simulink model "simplified_inverter"  (R2021b)
settings: Solver=ode23tb  StartTime=0.0  StopTime=0.1  MaxStep=10e-6  RelTol=1e-3  EnableMultiTasking=on
libraries: spsVoltageMeasurementLib x9, spsSeriesRLCBranchLib x6, spsControlledVoltageSourceLib x3, spsCurrentMeasurementLib x3, spsThreePhaseSourceLib x1, spspowerguiLib x1
settings Model: Creator=Алексей  LastModifiedBy=alexey
settings SolverCC: ZeroCrossControl=DisableAll  ZeroCrossAlgorithm=Adaptive  AlgebraicLoopSolver=TrustRegion
settings DataIOCC: SaveFormat=Array  SaveOutput=off  SignalLogging=off  DSMLogging=off  SaveTime=off  ReturnWorkspaceOutputs=off
settings OptimizationCC: LifeSpan=inf
settings DebuggingCC: UnderspecifiedInitializationDetection=Classic  MergeDetectMultiDrivingBlocksExec=none  SolverPrmCheckMsg=warning  AllowSymbolicDim=off  SFUnexpectedBacktrackingDiag=warning  SFNoUnconditionalDefaultTransitionDiag=warning  SFExecutionAtInitializationDiag=none  SFMachineParentedDataDiag=warning  ArithmeticOperatorsInVariantConditions=warning
settings HardwareCC: ProdBitPerPointer=32  ProdBitPerSizeT=32  ProdBitPerPtrDiffT=32  ProdLargestAtomicFloat=None  ProdIntDivRoundTo=Undefined  ProdEndianess=Unspecified  ProdWordSize=32  ProdHWDeviceType=32-bit Generic
settings ModelReferenceCC: PropagateSignalLabelsOutOfModel=off
settings SFSimCC: SimUseLocalCustomCode=off  CustomCodeUndefinedFunction=UseInterfaceOnly
settings RTWCC: RTWUseLocalCustomCode=off
settings CodeAppCC: StateflowObjectComments=on
settings GRTTargetCC: TargetLangStandard=C89/C90 (ANSI)  RTWCAPISignals=on  RTWCAPIParams=on
settings ConfigComp: CovMetricSettings=dw  CovSaveCumulativeToWorkspaceVar=on  CovSaveSingleToWorkspaceVar=on  CovExternalEMLEnable=off  CovSFcnEnable=off
settings SimscapeCC: SimscapeNormalizeSystem=off

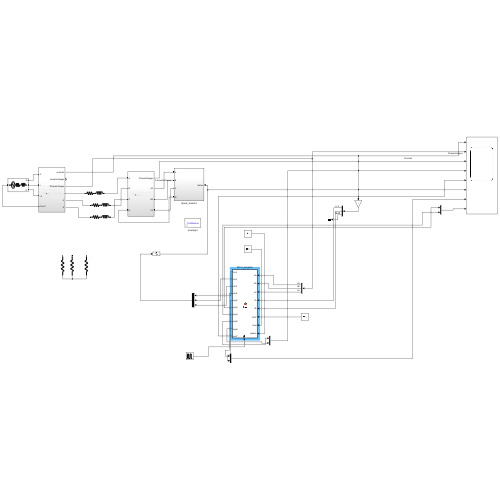
[thumbnail: Simulink's stored preview of the top-level diagram]
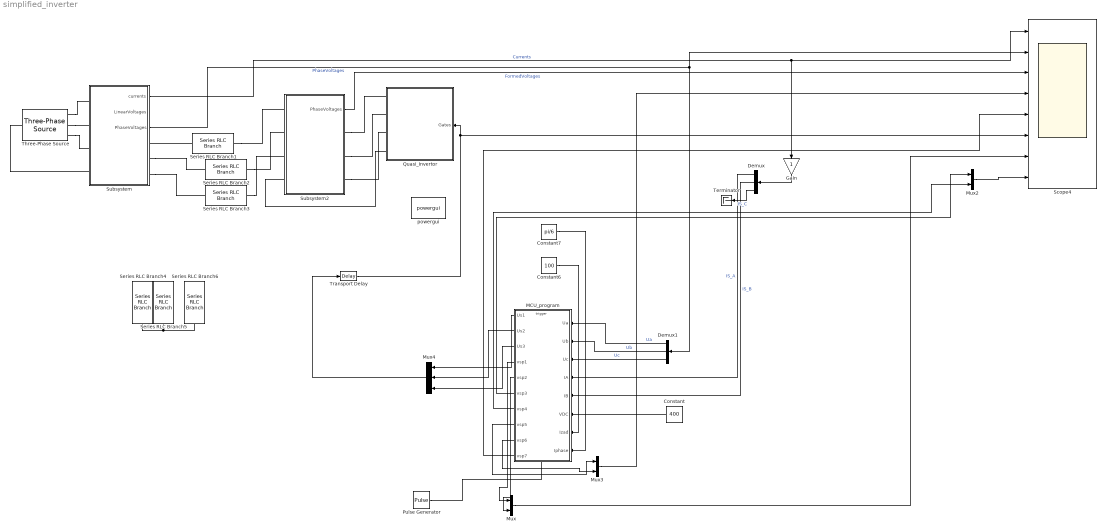
== system simplified_inverter ==
  Constant : Constant  Value=400
  Constant6 : Constant  Value=100
  Constant7 : Constant  Value=pi/6
  Demux : Demux  Outputs=3
  Demux1 : Demux  Outputs=3
  Gain : Gain
  MCU_program : MATLAB Function  TreatAsAtomicUnit=on
  Mux : Mux  Inputs=2
  Mux2 : Mux  Inputs=2
  Mux3 : Mux  Inputs=2
  Mux4 : Mux  Inputs=3
  Pulse Generator : DiscretePulseGenerator  PulseType=Time based  Period=10e-6  PulseWidth=10
  Quasi_Invertor : Subsystem
  Scope4 : Scope  NumInputPorts=8
  Series RLC Branch1 : spsSeriesRLCBranchLib/Series RLC Branch  LConnTagsString=__new0  RConnTagsString=__new0  BranchType=RL  Resistance=0.01  Inductance=50e-6  SetiL0=off  InitialCurrent=0  Capacitance=1e-6  Setx0=off  InitialVoltage=0  Measurements=None
  Series RLC Branch2 : spsSeriesRLCBranchLib/Series RLC Branch  LConnTagsString=__new0  RConnTagsString=__new0  BranchType=RL  Resistance=0.01  Inductance=50e-6  SetiL0=off  InitialCurrent=0  Capacitance=1e-6  Setx0=off  InitialVoltage=0  Measurements=None
  Series RLC Branch3 : spsSeriesRLCBranchLib/Series RLC Branch  LConnTagsString=__new0  RConnTagsString=__new0  BranchType=RL  Resistance=0.01  Inductance=50e-6  SetiL0=off  InitialCurrent=0  Capacitance=1e-6  Setx0=off  InitialVoltage=0  Measurements=None
  Series RLC Branch4 : spsSeriesRLCBranchLib/Series RLC Branch  LConnTagsString=__new0  RConnTagsString=__new0  BranchType=R  Resistance=10  Inductance=500e-6  SetiL0=off  InitialCurrent=0  Capacitance=1e-6  Setx0=off  InitialVoltage=0  Measurements=None
  Series RLC Branch5 : spsSeriesRLCBranchLib/Series RLC Branch  LConnTagsString=__new0  RConnTagsString=__new0  BranchType=R  Resistance=10  Inductance=500e-6  SetiL0=off  InitialCurrent=0  Capacitance=1e-6  Setx0=off  InitialVoltage=0  Measurements=None
  Series RLC Branch6 : spsSeriesRLCBranchLib/Series RLC Branch  LConnTagsString=__new0  RConnTagsString=__new0  BranchType=R  Resistance=10  Inductance=500e-6  SetiL0=off  InitialCurrent=0  Capacitance=1e-6  Setx0=off  InitialVoltage=0  Measurements=None
  Subsystem : Subsystem
  Subsystem2 : Subsystem
  Terminator : Terminator
  Three-Phase Source : spsThreePhaseSourceLib/Three-Phase Source  InternalConnection=Yn  VoltagePhases=on  Voltage=200  PhaseAngle=0  Voltage_phases=[200 200 200]/sqrt(2)  PhaseAngles_phases=[0 -120 +120]  Frequency=500  NonIdealSource=on  SpecifyImpedance=off  Resistance=1e-6  Inductance=30e-9  ShortCircuitLevel=100e6  BaseVoltage=200  XRratio=7  BusType=swing  Pref=10e3  Qref=0  Prefabc=[10e3, 10e3, 10e3]  Qrefabc=[0, 0, 0]  Qmin=-inf  Qmax=inf
  Transport Delay : TransportDelay  DelayTime=1e-6
  powergui : spspowerguiLib/powergui  Priority=1  SimulationMode=Continuous  SampleTime=50e-6  frequency=60  Iterations=50  frequencyindice=500  Pbase=100e6  ErrMax=1e-4  UnitsV=kV  UnitsW=MW  buscounter=0  FunctionMessages=off  echomessages=off  EnableUseOfTLC=off  CurrentSourceSwitches=on  DisableSnubberDevices=off  DisableRonSwitches=off  DisableVfSwitches=off  DisplayEquations=off  AutomaticDiscreteSolvers=off  SolverType=Tustin  Interpol=off  ExternalGateDelay=off  methode=off  Ts=0  x0status=zero  SPID=off  SwTol=0  HookPort=off  NonlinearTolerance=1e-4  nMaxIteration=100  ContinueOnMaxIteration=off  RestoreLinks=warning  ResistiveCurrentMeasurement=off  Frange=[0:2:500]  Ylog=off  Xlog=on  ShowGrid=off  save=off  variable=ZData  structure=SD2  ZoomFFT=on  StartTime=0.7  cycles=10  DisplayStyle=4  fundamental=382  FreqAxis=off  MaxFrequency=50000  frequencyindicesteady=1  RmsSteady=1  display=off
  wires:
  Demux/1 -> MCU_program/4(IA)  "IS_A"
  Demux/2 -> MCU_program/5(IB)  "IS_B"
  MCU_program/5(vsp2) -> Mux/2
  MCU_program/4(vsp1) -> Mux/1
  MCU_program/3(Us3) -> Mux4/3
  Mux4/1 -> Transport Delay/1
  MCU_program/1(Us1) -> Mux4/1
  Pulse Generator/1 -> MCU_program/Trigger
  MCU_program/2(Us2) -> Mux4/2
  Demux/3 -> Terminator/1  "IS_C"
  Demux1/1 -> MCU_program/1(Ua)  "Ua"
  Demux1/2 -> MCU_program/2(Ub)  "Ub"
  Demux1/3 -> MCU_program/3(Uc)  "Uc"
  Subsystem/1(currents) -> Gain/1, Scope4/1  "Currents"
  Mux/1 -> Scope4/7
  Subsystem/3(PhaseVoltages) -> Scope4/2, Demux1/1  "PhaseVoltages"
  MCU_program/7(vsp4) -> Mux2/2
  Constant6/1 -> MCU_program/7(Izad)
  Constant7/1 -> MCU_program/8(Iphase)
  Mux2/1 -> Scope4/8
  MCU_program/6(vsp3) -> Mux2/1
  MCU_program/8(vsp5) -> Mux3/1
  MCU_program/9(vsp6) -> Mux3/2
  Mux3/1 -> Scope4/4
  MCU_program/10(vsp7) -> Scope4/5
  Gain/1 -> Demux/1
  Transport Delay/1 -> Scope4/6, Quasi_Invertor/1(Gates)
  Subsystem2/1(PhaseVoltages) -> Scope4/3  "FormedVoltages"
  Constant/1 -> MCU_program/6(VDC)
  connections:
  Three-Phase Source/RConn1 -- Subsystem/LConn1
  Three-Phase Source/RConn2 -- Subsystem/LConn2
  Three-Phase Source/RConn3 -- Subsystem/LConn3
  Series RLC Branch1/RConn1 -- Subsystem2/LConn1
  Three-Phase Source/LConn1 -- Subsystem/LConn4
  Subsystem2/RConn1 -- Quasi_Invertor/RConn1
  Subsystem2/RConn2 -- Quasi_Invertor/RConn2
  Subsystem2/RConn3 -- Quasi_Invertor/RConn3
  Series RLC Branch2/RConn1 -- Subsystem2/LConn2
  Series RLC Branch3/RConn1 -- Subsystem2/LConn3
  Subsystem2/LConn4 -- Quasi_Invertor/RConn4
  Series RLC Branch4/RConn1 -- Series RLC Branch6/RConn1 -- Series RLC Branch5/RConn1
  Series RLC Branch1/LConn1 -- Subsystem/RConn1
  Subsystem/RConn2 -- Series RLC Branch2/LConn1
  Subsystem/RConn3 -- Series RLC Branch3/LConn1

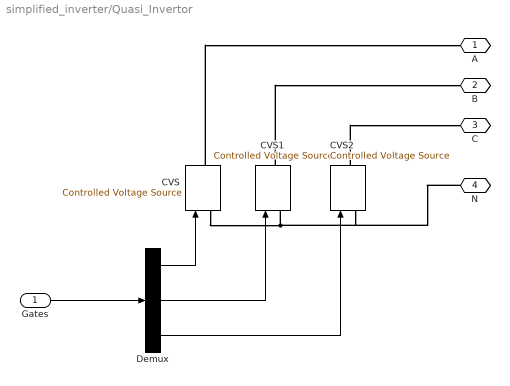
== system simplified_inverter/Quasi_Invertor ==
  Gates : Inport
  CVS : spsControlledVoltageSourceLib/Controlled Voltage Source  Initialize=on  Source_Type=AC  Amplitude=0  Phase=0  Frequency=0  Measurements=None
  CVS1 : spsControlledVoltageSourceLib/Controlled Voltage Source  Initialize=on  Source_Type=AC  Amplitude=0  Phase=0  Frequency=0  Measurements=None
  CVS2 : spsControlledVoltageSourceLib/Controlled Voltage Source  Initialize=on  Source_Type=AC  Amplitude=0  Phase=0  Frequency=0  Measurements=None
  Demux : Demux  Outputs=3
  A : PMIOPort  Side=Right
  B : PMIOPort  Port=2  Side=Right
  C : PMIOPort  Port=3  Side=Right
  N : PMIOPort  Port=4  Side=Right
  wires:
  Demux/1 -> CVS/1
  Demux/2 -> CVS1/1
  Demux/3 -> CVS2/1
  Gates/1 -> Demux/1
  connections:
  CVS1/RConn1 -- B/RConn1
  CVS2/RConn1 -- C/RConn1
  CVS/RConn1 -- A/RConn1
  CVS/LConn1 -- N/RConn1 -- CVS2/LConn1 -- CVS1/LConn1

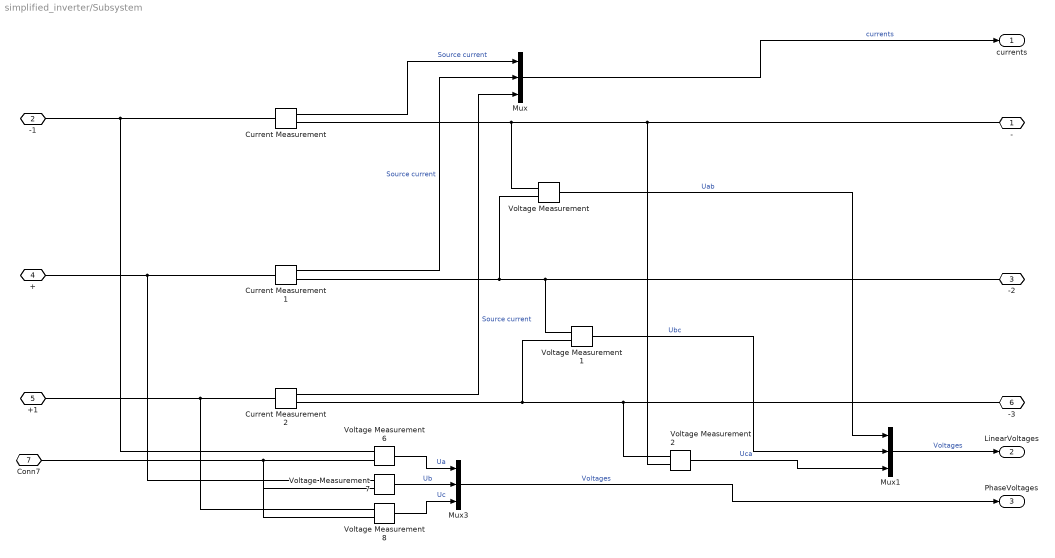
== system simplified_inverter/Subsystem ==
  Current Measurement : spsCurrentMeasurementLib/Current Measurement  PhasorSimulation=off  OutputType=Complex  PSBequivalent=0
  Current Measurement1 : spsCurrentMeasurementLib/Current Measurement  PhasorSimulation=off  OutputType=Complex  PSBequivalent=0
  Current Measurement2 : spsCurrentMeasurementLib/Current Measurement  PhasorSimulation=off  OutputType=Complex  PSBequivalent=0
  Mux : Mux  Inputs=3
  Mux1 : Mux  Inputs=3
  Mux3 : Mux  Inputs=3
  Voltage Measurement{,1..2,6..8} (6 alike) : spsVoltageMeasurementLib/Voltage Measurement  PhasorSimulation=off  OutputType=Complex  PSBequivalent=0
  - : PMIOPort  Side=Right
  -1 : PMIOPort  Port=2  Side=Left
  -2 : PMIOPort  Port=3  Side=Right
  + : PMIOPort  Port=4  Side=Left
  +1 : PMIOPort  Port=5  Side=Left
  -3 : PMIOPort  Port=6  Side=Right
  Conn7 : PMIOPort  Port=7  Side=Left
  currents : Outport
  LinearVoltages : Outport  Port=2
  PhaseVoltages : Outport  Port=3
  wires:
  Current Measurement2/1 -> Mux/3  "Source current"
  Current Measurement1/1 -> Mux/2  "Source current"
  Voltage Measurement1/1 -> Mux1/2  "Ubc"
  Voltage Measurement2/1 -> Mux1/3  "Uca"
  Mux/1 -> currents/1  "currents"
  Voltage Measurement/1 -> Mux1/1  "Uab"
  Current Measurement/1 -> Mux/1  "Source current"
  Mux1/1 -> LinearVoltages/1  "Voltages"
  Mux3/1 -> PhaseVoltages/1  "Voltages"
  Voltage Measurement8/1 -> Mux3/3  "Uc"
  Voltage Measurement6/1 -> Mux3/1  "Ua"
  Voltage Measurement7/1 -> Mux3/2  "Ub"
  connections:
  -1/RConn1 -- Voltage Measurement6/LConn1 -- Current Measurement/LConn1
  Current Measurement1/RConn1 -- Voltage Measurement/LConn2 -- -2/RConn1 -- Voltage Measurement1/LConn1
  Current Measurement/RConn1 -- Voltage Measurement/LConn1 -- Voltage Measurement2/LConn2 -- -/RConn1
  Current Measurement2/RConn1 -- Voltage Measurement2/LConn1 -- -3/RConn1 -- Voltage Measurement1/LConn2
  Voltage Measurement6/LConn2 -- Voltage Measurement8/LConn2 -- Voltage Measurement7/LConn2 -- Conn7/RConn1
  +1/RConn1 -- Voltage Measurement8/LConn1 -- Current Measurement2/LConn1
  +/RConn1 -- Voltage Measurement7/LConn1 -- Current Measurement1/LConn1

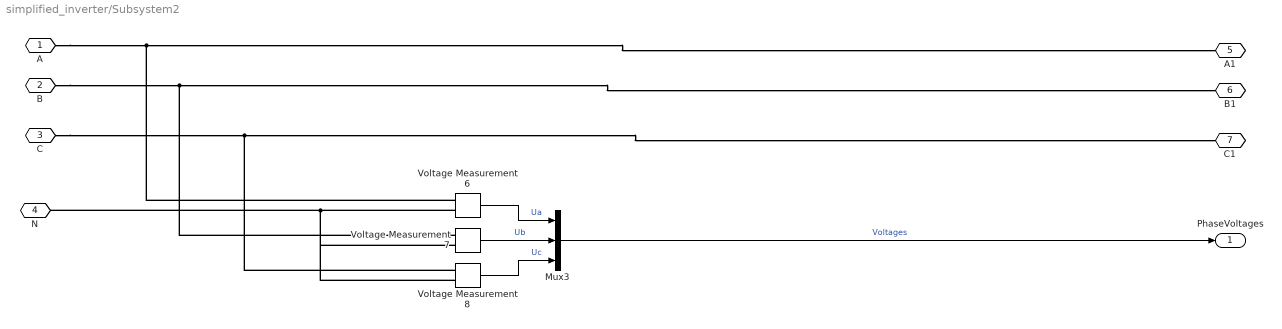
== system simplified_inverter/Subsystem2 ==
  Mux3 : Mux  Inputs=3
  Voltage Measurement6 : spsVoltageMeasurementLib/Voltage Measurement  PhasorSimulation=off  OutputType=Complex  PSBequivalent=0
  Voltage Measurement7 : spsVoltageMeasurementLib/Voltage Measurement  PhasorSimulation=off  OutputType=Complex  PSBequivalent=0
  Voltage Measurement8 : spsVoltageMeasurementLib/Voltage Measurement  PhasorSimulation=off  OutputType=Complex  PSBequivalent=0
  A : PMIOPort  Side=Left
  B : PMIOPort  Port=2  Side=Left
  C : PMIOPort  Port=3  Side=Left
  N : PMIOPort  Port=4  Side=Left
  A1 : PMIOPort  Port=5  Side=Right
  B1 : PMIOPort  Port=6  Side=Right
  C1 : PMIOPort  Port=7  Side=Right
  PhaseVoltages : Outport
  wires:
  Voltage Measurement7/1 -> Mux3/2  "Ub"
  Voltage Measurement6/1 -> Mux3/1  "Ua"
  Voltage Measurement8/1 -> Mux3/3  "Uc"
  Mux3/1 -> PhaseVoltages/1  "Voltages"
  connections:
  Voltage Measurement7/LConn2 -- Voltage Measurement8/LConn2 -- Voltage Measurement6/LConn2 -- N/RConn1
  Voltage Measurement8/LConn1 -- C1/RConn1 -- C/RConn1
  Voltage Measurement6/LConn1 -- A1/RConn1 -- A/RConn1
  Voltage Measurement7/LConn1 -- B1/RConn1 -- B/RConn1

== matlab function simplified_inverter/MCU_program ==
  data: Ua input; Ub input; Uc input; IA input; IB input; Us1 output; Us2 output; Us3 output; vsp1 output; vsp2 output; vsp3 output; vsp4 output; VDC input; Izad input; Iphase input; vsp5 output; vsp6 output; vsp7 output
  events: trigger input RISING_EDGE_EVENT
function [Us1,Us2,Us3,vsp1,vsp2,vsp3,vsp4,vsp5,vsp6,vsp7] = fcn(Ua,Ub,Uc,IA,IB,VDC, Izad, Iphase)
%время 1/2 ШИМ периода
dt = 10e-6;

kuqp = 10;
kuqi = 1000;

kudp = 10;
kudi = 1000;






persistent Uqint;
if isempty(Uqint)
    Uqint=0;
end 
persistent Udint;
if isempty(Udint)
    Udint=0;
end 


Ialfa = -IA;
Ibeta = -(2*IB+IA)/sqrt(3);
I_ampl = sqrt(Ialfa^2+Ibeta^2);

Ualfa = Ua;
Ubeta = (2*Ub+Ua)/sqrt(3);

U_ampl = sqrt(Ualfa^2+Ubeta^2);
teta=acos(Ualfa/U_ampl)*sign(Ubeta)+(sign(Ubeta)-1)*(-pi);



%реальные значения токов Id и Iq, полученные через  угол и оси альфа,бета 
Iact = Ialfa*cos(teta)+Ibeta*sin(teta);
Iact = -Iact; %Перевод в систему координат инвертора - для него поглощается активный ток сети
Ireact = Ibeta*cos(teta)-Ialfa*sin(teta); 

Ireact_zad = -Izad * sin(Iphase);
%ПИ-регулятор для напряжения по оси Ку
direact = Ireact_zad-Ireact;
Uqpr = direact*kuqp;
Uqint=Uqint+direact*kuqi*dt;


Iact_zad = Izad * cos(Iphase);
%ПИ-регулятор для напряжения по оси Дэ
diact = Iact_zad-Iact;
Udpr = diact*kudp;
Udint=Udint+diact*kudi*dt;

Um = (2/3)*VDC/sqrt(Uqpr^2+Udpr^2)*0.85;

if(Um<1)
  Uqpr = Uqpr*Um;
  Udpr = Udpr*Um;
end

  
U_q=Uqpr+Uqint;                    
U_d=Udpr+Udint;


%U_q = 0;
U_d = -U_d;



Ua0=U_d*cos(teta)-U_q*sin(teta);
Ub0=U_d*sin(teta)+U_q*cos(teta);
vrefa=sqrt(Ua0^2+Ub0^2);
tetaV = acos(Ua0/vrefa)*sign(Ub0)+(sign(Ub0)-1)*(-pi);

vsp1=Ualfa;
vsp2=Ua0;
vsp3=Ubeta;
vsp4=Ub0;
vsp5 = Iact;
vsp6 = Ireact;
vsp7 = teta;



%алгоритм формирования фазных напряжений, КЛАРК


Us1=ceil(Ua0*100)/100;
Us2=sqrt(3)/2*Ub0-0.5*Ua0;
Us2=ceil(Us2*100)/100;
Us3=-0.5*Ua0-sqrt(3)/2*Ub0;
Us3=ceil(Us3*100)/100;
return;
